simulink model "simu_gimbal"  (R2020a)
settings: Solver=FixedStepAuto  StartTime=0.0  StopTime=20  FixedStep=0.002  RelTol=1e-3
InitFcn:
  | init_conditions
values from neighbouring files (symbols this model uses):
  a = 1    [init_conditions.m]
  B = 0    [init_conditions.m]
  IB = diag([IBxy, IBxy, IBz])    [init_conditions.m]
  Iz = 3*(10^-5)    (= 3e-05)    [init_conditions.m]
  K = 0    [init_conditions.m]
  K1 = 800    [init_conditions.m]
  Lh = [0;0;0]    [init_conditions.m]
  m = (m_qc+0.006)*4 + m_main    (= 0.156)    [init_conditions.m]
  m_main = 0.012    [init_conditions.m]
undefined symbols (not defined in the file or in its folder): X, Y, Z
libraries: nesl_utility x25, sm_lib x24, sharedtransform x3, simulink x2
settings Model: Creator=Paul  LastModifiedBy=lee
settings DataIOCC: ReturnWorkspaceOutputs=off
settings DebuggingCC: ArithmeticOperatorsInVariantConditions=warning
settings SFSimCC: SimUseLocalCustomCode=off  CustomCodeUndefinedFunction=UseInterfaceOnly
settings RTWCC: RTWUseLocalCustomCode=off
settings ExplorerConfigSet: InternalSimMechanicsExplorerSettings="<ExplorerConfiguration><canonicalview>default</canonicalview><AnimationSetting><BasePlaybackSpeed>1.0</BasePlaybackSpeed><PlaybackSpeedFactor>1.0</PlaybackSpeedFactor></AnimationSetting><TilePanel><TileInfo><Tiles Columns=\"1\" Count=\"1\" Rows=\"1\"><Column Weight=\"1\"/><Row Weight=\"1\"/><Tile Height=\"1\" Width=\"1\" X=\"0\" Y=\"0\"/></Tiles></TileInfo><SceneInfo><SceneViewer><BGColor><R>0.60000002384185791</R><G>0.60000002384185791</G><B>0.60000002384185791</B></BGColor><Camera><DoPerspective>off</DoPerspective><Position><X>0.105450656144933763</X><Y>-0.11353615296204797</Y><Z>1.90562556726929944</Z></Position><Center><X>0.163716647023041978</X><Y>-0.0279701005319462764</Y><Z>-0.924535797346482835</Z></Center><Up><X>0.999736240990410918</X><Y>-0.0108255212991936745</Y><Z>0.0202547905189051844</Z></Up><ViewLimDist>1</ViewLimDist><YLim>0.670906463981186918</YLim><XLim>0.633335701998240408</XLim></Camera></SceneViewer></SceneInfo></TilePanel><MechEditorPanel><Cameras/><GfxPanelCameraMap/><VideoCreator><PlaybackSpeedRatio>1.0</PlaybackSpeedRatio><FrameRate>30</FrameRate><VideoFormat>Motion JPEG AVI</VideoFormat><FrameSize>auto</FrameSize></VideoCreator></MechEditorPanel></ExplorerConfiguration>"

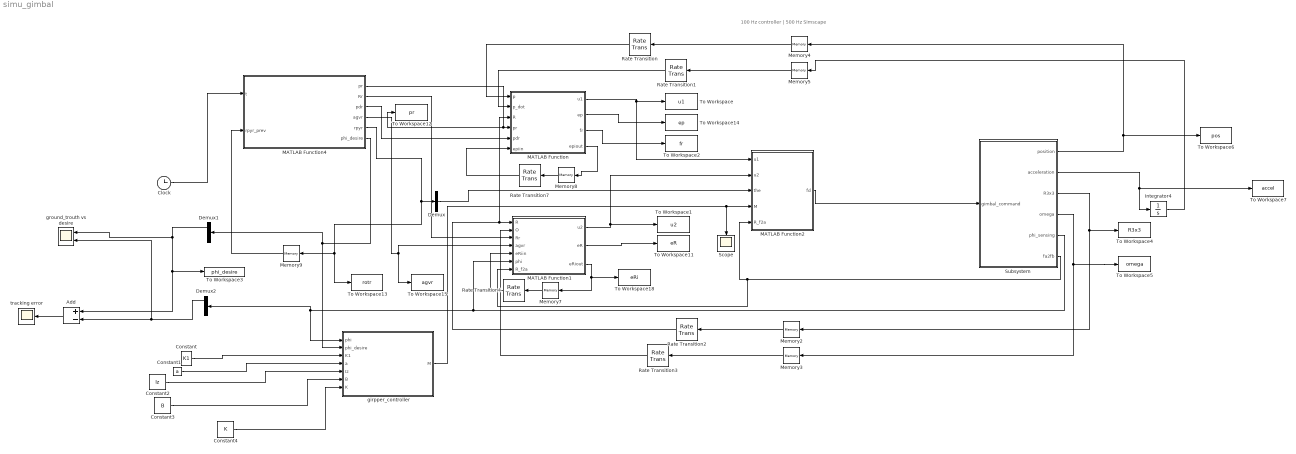
== system simu_gimbal ==
  note: 100 Hz controller | 500 Hz Simscape
  Add : Sum  Inputs=+-
  Clock : Clock
  Constant : Constant  Value=K1
  Constant1 : Constant  Value=a
  Constant2 : Constant  Value=Iz
  Constant3 : Constant  Value=B
  Constant4 : Constant  Value=K
  Demux : Demux  Outputs=3
  Demux1 : Demux  Outputs=3
  Demux2 : Demux  Outputs=3
  Integrator4 : Integrator  InitialCondition=[0;0;0]
  MATLAB Function : MATLAB Function  TreatAsAtomicUnit=on
  MATLAB Function1 : MATLAB Function  TreatAsAtomicUnit=on
  MATLAB Function2 : MATLAB Function  TreatAsAtomicUnit=on
  MATLAB Function4 : MATLAB Function  TreatAsAtomicUnit=on
  Memory2 : Memory  InitialCondition=eye(3)
  Memory{3..5,7..9} (6 alike) : Memory  InitialCondition=[0;0;0]
  Rate Transition{,1..4,7} (6 alike) : RateTransition  OutPortSampleTime=0.01
  Scope : Scope
  Subsystem : Subsystem
  To Workspace : ToWorkspace  VariableName=u1  SaveFormat=Timeseries  SampleTime=-1
  To Workspace1 : ToWorkspace  VariableName=u2  SaveFormat=Timeseries  SampleTime=-1
  To Workspace11 : ToWorkspace  VariableName=eR  SaveFormat=Timeseries  SampleTime=-1
  To Workspace12 : ToWorkspace  VariableName=pr  SaveFormat=Timeseries  SampleTime=-1
  To Workspace13 : ToWorkspace  VariableName=rotr  SaveFormat=Timeseries  SampleTime=-1
  To Workspace14 : ToWorkspace  VariableName=ep  SaveFormat=Timeseries  SampleTime=-1
  To Workspace15 : ToWorkspace  VariableName=agvr  SaveFormat=Timeseries  SampleTime=-1
  To Workspace18 : ToWorkspace  VariableName=eRi  SaveFormat=Timeseries  SampleTime=-1
  To Workspace2 : ToWorkspace  VariableName=fr  SaveFormat=Timeseries  SampleTime=-1
  To Workspace3 : ToWorkspace  VariableName=phi_desire  SaveFormat=Timeseries  SampleTime=-1
  To Workspace4 : ToWorkspace  VariableName=R3x3  SaveFormat=Timeseries  SampleTime=-1
  To Workspace5 : ToWorkspace  VariableName=omega  SaveFormat=Timeseries  SampleTime=-1
  To Workspace6 : ToWorkspace  VariableName=pos  SaveFormat=Timeseries  SampleTime=-1
  To Workspace7 : ToWorkspace  VariableName=accel  SaveFormat=Timeseries  SampleTime=-1
  girpper_controller : MATLAB Function  TreatAsAtomicUnit=on
  ground_trouth vs desire : Scope  NumInputPorts=2
  tracking error : Scope
  wires:
  MATLAB Function/1(u1) -> MATLAB Function2/1(u1), To Workspace/1
  MATLAB Function1/1(u2) -> MATLAB Function2/2(u2), To Workspace1/1
  Subsystem/3(R3x3) -> To Workspace4/1, Memory2/1
  Memory2/1 -> Rate Transition2/1
  Subsystem/4(omega) -> To Workspace5/1, Memory3/1
  Memory3/1 -> Rate Transition3/1
  Memory4/1 -> Rate Transition/1
  Memory5/1 -> Rate Transition1/1
  Subsystem/1(position) -> Memory4/1, To Workspace6/1
  Subsystem/2(acceleration) -> To Workspace7/1, Integrator4/1
  Integrator4/1 -> Memory5/1
  Clock/1 -> MATLAB Function4/1(t)
  MATLAB Function4/1(pr) -> To Workspace12/1, MATLAB Function/4(pr)
  MATLAB Function4/2(Rr) -> MATLAB Function1/3(Rr)
  MATLAB Function/3(fr) -> To Workspace2/1
  MATLAB Function2/1(fd) -> Subsystem/1(gimbal_command)
  MATLAB Function1/2(eR) -> To Workspace11/1
  MATLAB Function/2(ep) -> To Workspace14/1
  MATLAB Function1/3(eRiout) -> To Workspace18/1, Memory7/1
  Rate Transition/1 -> MATLAB Function/1(p)
  Rate Transition1/1 -> MATLAB Function/2(p_dot)
  Rate Transition2/1 -> MATLAB Function1/1(R), MATLAB Function/3(R)
  Rate Transition3/1 -> MATLAB Function1/2(O)
  Memory7/1 -> Rate Transition4/1
  Rate Transition4/1 -> MATLAB Function1/5(eRiin)
  Memory8/1 -> Rate Transition7/1
  MATLAB Function/4(epiout) -> Memory8/1
  Rate Transition7/1 -> MATLAB Function/6(epiin)
  MATLAB Function4/3(pdr) -> MATLAB Function/5(pdr)
  MATLAB Function4/4(agvr) -> To Workspace15/1, MATLAB Function1/4(agvr)
  MATLAB Function4/5(rpyr) -> To Workspace13/1, Memory9/1, Demux/1
  Memory9/1 -> MATLAB Function4/2(rpyr_prev)
  Demux/2 -> MATLAB Function2/3(the)
  Subsystem/5(phi_sensing) -> MATLAB Function1/6(phi), girpper_controller/1(phi), Demux2/1
  MATLAB Function4/6(phi_desire) -> Demux1/1, girpper_controller/2(phi_desire)
  Constant/1 -> girpper_controller/3(K1)
  Constant1/1 -> girpper_controller/4(a)
  girpper_controller/1(M) -> Scope/1, MATLAB Function2/4(M)
  Add/1 -> tracking error/1
  Demux1/1 -> To Workspace3/1, Add/1, ground_trouth vs desire/1
  Demux2/1 -> ground_trouth vs desire/2, Add/2
  Constant2/1 -> girpper_controller/5(Iz)
  Constant3/1 -> girpper_controller/6(B)
  Constant4/1 -> girpper_controller/7(K)
  Subsystem/6(fa2fb) -> MATLAB Function1/7(R_f2a), MATLAB Function2/5(R_f2a)

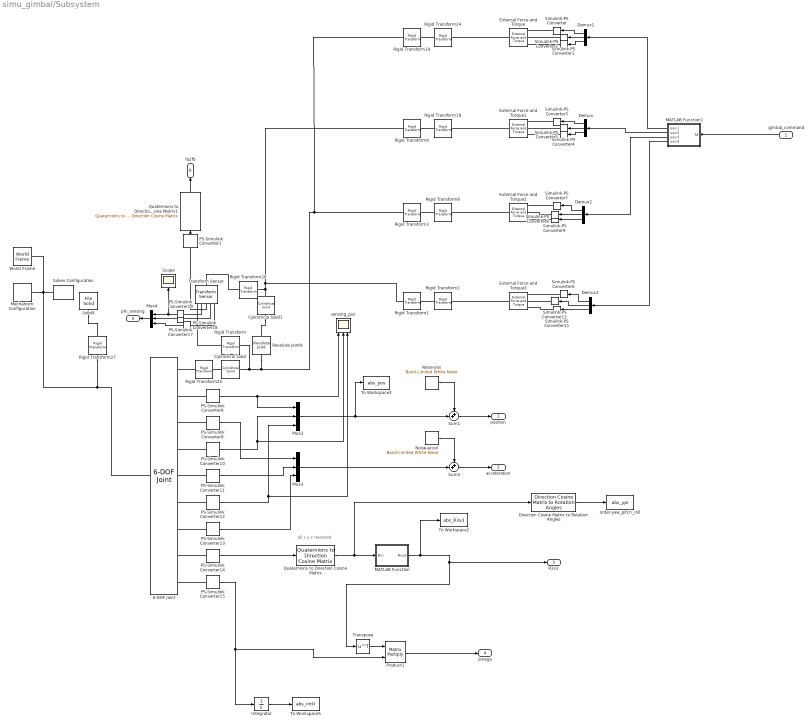
== system simu_gimbal/Subsystem ==
  note: all x y z reversed
  gimbal_command : Inport
  6-DOF Joint : sm_lib/Joints/6-DOF Joint  JointMode=Normal  SenseConstraintForce=off  SenseConstraintForceX=off  SenseConstraintForceY=off  SenseConstraintForceZ=off  SenseConstraintTorque=off  SenseConstraintTorqueX=off  SenseConstraintTorqueY=off  SenseConstraintTorqueZ=off  SenseTotalForce=off  SenseTotalForceX=off  SenseTotalForceY=off  SenseTotalForceZ=off  SenseTotalTorque=off  SenseTotalTorqueX=off  SenseTotalTorqueY=off  SenseTotalTorqueZ=off  CompositeWrenchDir=FollowerOnBase  CompositeWrenchFrame=BaseFrame  PxEquilibriumPosition=0  PxEquilibriumPositionUnits=m  PxSpringStiffness=0  PxSpringStiffnessUnits=N/m  PxDampingCoefficient=0  PxDampingCoefficientUnits=N/(m/s)  PxTorqueActuationMode=NoTorque  PxMotionActuationMode=ComputedMotion  PxSensePosition=on  PxSenseVelocity=off  PxSenseAcceleration=on  PxSenseTorqueForce=off  PxSenseLowerLimitTorqueForce=off  PxSenseUpperLimitTorqueForce=off  PxLowerLimitSpecify=off  PxLowerLimitBound=-1  PxLowerLimitBoundUnits=m  PxLowerLimitStiffness=1e6  PxLowerLimitStiffnessUnits=N/m  PxLowerLimitDamping=1e3  PxLowerLimitDampingUnits=N/(m/s)  PxLowerLimitTransitionRegionWidth=1e-4  PxLowerLimitTransitionRegionWidthUnits=m  PxUpperLimitSpecify=off  PxUpperLimitBound=1  PxUpperLimitBoundUnits=m  PxUpperLimitStiffness=1e6  PxUpperLimitStiffnessUnits=N/m  PxUpperLimitDamping=1e3  PxUpperLimitDampingUnits=N/(m/s)  PxUpperLimitTransitionRegionWidth=1e-4  PxUpperLimitTransitionRegionWidthUnits=m  PxPositionTargetSpecify=off  PxPositionTargetPriority=High  PxPositionTargetValue=0  PxPositionTargetValueUnits=m  PxVelocityTargetSpecify=off  PxVelocityTargetPriority=High  PxVelocityTargetValue=0  PxVelocityTargetValueUnits=m/s  PyEquilibriumPosition=0  PyEquilibriumPositionUnits=m  PySpringStiffness=0  PySpringStiffnessUnits=N/m  PyDampingCoefficient=0  PyDampingCoefficientUnits=N/(m/s)  PyTorqueActuationMode=NoTorque  PyMotionActuationMode=ComputedMotion  PySensePosition=on  PySenseVelocity=off  PySenseAcceleration=on  PySenseTorqueForce=off  PySenseLowerLimitTorqueForce=off  PySenseUpperLimitTorqueForce=off  PyLowerLimitSpecify=off  PyLowerLimitBound=-1  PyLowerLimitBoundUnits=m  PyLowerLimitStiffness=1e6  PyLowerLimitStiffnessUnits=N/m  PyLowerLimitDamping=1e3  PyLowerLimitDampingUnits=N/(m/s)  PyLowerLimitTransitionRegionWidth=1e-4  PyLowerLimitTransitionRegionWidthUnits=m  PyUpperLimitSpecify=off  PyUpperLimitBound=1  PyUpperLimitBoundUnits=m  PyUpperLimitStiffness=1e6  PyUpperLimitStiffnessUnits=N/m  PyUpperLimitDamping=1e3  PyUpperLimitDampingUnits=N/(m/s)  PyUpperLimitTransitionRegionWidth=1e-4  PyUpperLimitTransitionRegionWidthUnits=m  PyPositionTargetSpecify=off  PyPositionTargetPriority=High  PyPositionTargetValue=0  PyPositionTargetValueUnits=m  PyVelocityTargetSpecify=off  PyVelocityTargetPriority=High  PyVelocityTargetValue=0  PyVelocityTargetValueUnits=m/s  PzEquilibriumPosition=0  PzEquilibriumPositionUnits=m  PzSpringStiffness=0  PzSpringStiffnessUnits=N/m  PzDampingCoefficient=0  PzDampingCoefficientUnits=N/(m/s)  PzTorqueActuationMode=NoTorque  PzMotionActuationMode=ComputedMotion  PzSensePosition=on  PzSenseVelocity=off  PzSenseAcceleration=on  PzSenseTorqueForce=off  PzSenseLowerLimitTorqueForce=off  PzSenseUpperLimitTorqueForce=off  PzLowerLimitSpecify=off  PzLowerLimitBound=-1  PzLowerLimitBoundUnits=m  PzLowerLimitStiffness=1e6  PzLowerLimitStiffnessUnits=N/m  PzLowerLimitDamping=1e3  PzLowerLimitDampingUnits=N/(m/s)  PzLowerLimitTransitionRegionWidth=1e-4  PzLowerLimitTransitionRegionWidthUnits=m  PzUpperLimitSpecify=off  PzUpperLimitBound=1  PzUpperLimitBoundUnits=m  PzUpperLimitStiffness=1e6  PzUpperLimitStiffnessUnits=N/m  PzUpperLimitDamping=1e3  PzUpperLimitDampingUnits=N/(m/s)  PzUpperLimitTransitionRegionWidth=1e-4  PzUpperLimitTransitionRegionWidthUnits=m  PzPositionTargetSpecify=off  PzPositionTargetPriority=High  PzPositionTargetValue=0  PzPositionTargetValueUnits=m  PzVelocityTargetSpecify=off  PzVelocityTargetPriority=High  PzVelocityTargetValue=0  PzVelocityTargetValueUnits=m/s  SphDefPosRotationMethod=None  SphDefPosRotationAngleUnits=deg  SphDefPosRotationStandardAxis=+Z  SphDefPosRotationAngle=0.0  SphDefPosRotationArbitraryAxis=[0 0 1]  SphDefPosFollAlignAxisA=+X  SphDefPosBaseAlignAxisA=+Y  SphDefPosFollAlignAxisB=+Y  SphDefPosBaseAlignAxisB=+Z  SphDefPosRotationSequenceAxes=FollowerAxes  SphDefPosRotationSequence=XYX  SphDefPosRotationSequenceAngles=[0 0 0]  SphDefPosRotationSequenceAnglesUnits=deg  SphDefPosRotationMatrix=[1 0 0; 0 1 0; 0 0 1]  SphEqPosRotationMethod=None  SphEqPosRotationAngleUnits=deg  SphEqPosRotationStandardAxis=+Z  SphEqPosRotationAngle=0.0  SphEqPosRotationArbitraryAxis=[0 0 1]  SphEqPosFollAlignAxisA=+X  SphEqPosBaseAlignAxisA=+Y  SphEqPosFollAlignAxisB=+Y  SphEqPosBaseAlignAxisB=+Z  SphEqPosRotationSequenceAxes=FollowerAxes  SphEqPosRotationSequence=XYX  SphEqPosRotationSequenceAngles=[0 0 0]  SphEqPosRotationSequenceAnglesUnits=deg  SphEqPosRotationMatrix=[1 0 0; 0 1 0; 0 0 1]  SphSpringStiffness=0  SphSpringStiffnessUnits=N*m/deg  SphDampingCoefficient=0  SphDampingCoefficientUnits=N*m/(deg/s)  SphActuateTorqueX=off  SphActuateTorqueY=off  SphActuateTorqueZ=off  SphActuateTorque=off  SphTorqueActuationMode=NoTorque  SphMotionActuationMode=ComputedMotion  SphActuationFrame=BaseFrame  SphSensePosition=on  SphSenseVelocityX=off  SphSenseVelocityY=off  SphSenseVelocityZ=off  SphSenseVelocity=on  SphSenseAccelerationX=off  SphSenseAccelerationY=off  SphSenseAccelerationZ=off  SphSenseAcceleration=off  SphSenseTorqueX=off  SphSenseTorqueY=off  SphSenseTorqueZ=off  SphSenseTorqueForce=off  SphSenseLowerLimitTorqueMag=off  SphSenseUpperLimitTorqueMag=off  SphSensingFrame=BaseFrame  SphLowerLimitSpecify=off  SphLowerLimitBound=15  SphLowerLimitBoundUnits=deg  SphLowerLimitStiffness=1e4  SphLowerLimitStiffnessUnits=N*m/deg  SphLowerLimitDamping=10  SphLowerLimitDampingUnits=N*m/(deg/s)  SphLowerLimitTransitionRegionWidth=0.1  SphLowerLimitTransitionRegionWidthUnits=deg  SphUpperLimitSpecify=off  SphUpperLimitBound=45  SphUpperLimitBoundUnits=deg  SphUpperLimitStiffness=1e4  SphUpperLimitStiffnessUnits=N*m/deg  SphUpperLimitDamping=10  SphUpperLimitDampingUnits=N*m/(deg/s)  SphUpperLimitTransitionRegionWidth=0.1  SphUpperLimitTransitionRegionWidthUnits=deg  SphPositionTargetRotationMethod=None  SphPositionTargetRotationAngleUnits=deg  SphPositionTargetRotationStandardAxis=+Z  SphPositionTargetRotationAngle=0.0  SphPositionTargetRotationArbitraryAxis=[0 0 1]  SphPositionTargetFollAlignAxisA=+X  SphPositionTargetBaseAlignAxisA=+Y  SphPositionTargetFollAlignAxisB=+Y  SphPositionTargetBaseAlignAxisB=+Z  SphPositionTargetRotationSequenceAxes=FollowerAxes  SphPositionTargetRotationSequence=XYX  SphPositionTargetRotationSequenceAngles=[0 0 0]  SphPositionTargetRotationSequenceAnglesUnits=deg  SphPositionTargetRotationMatrix=[1 0 0; 0 1 0; 0 0 1]  SphPositionTargetSpecify=off  SphPositionTargetPriority=High  SphVelocityTargetValue=[0 0 0]  SphVelocityTargetValueUnits=deg/s  SphVelocityTargetSpecify=off  SphVelocityTargetPriority=High  SphVelocityTargetInFollowerFrame=on
  Cylindrical Solid : sm_lib/Body Elements/Cylindrical Solid  GraphicAmbientColor=[0.15 0.15 0.15 1.0]  BasedOnType=Density  CenterOfMass=[0 0 0]  CenterOfMassUnits=m  GraphicDiffuseColor=[0.5 0.5 0.5]  CylinderLength=300  CylinderLengthUnits=mm  CylinderRadius=3  CylinderRadiusUnits=mm  Density=1000  DensityUnits=kg/m^3  DoExposeReferenceFrame=off  GraphicEmissiveColor=[0.0 0.0 0.0 1.0]  ExportEntireGeometry=off  SerializedFrames=<Frames><Frame><Id>Frame1</Id><Value><Name>F1</Name><Origin><Source>ReferenceFrame</Source><FeatureName></FeatureName></Origin><PrimaryAxis><DefinedDirection>+Z</DefinedDirection><Source>ReferenceFrame</Source><SourceDirection>+Y</SourceDirection><FeatureName></FeatureName></PrimaryAxis><SecondaryAxis><DefinedDirection>+Y</DefinedDirection><Source>ReferenceFrame</Source><SourceDirection>+X</SourceDirection><FeatureName></FeatureName></SecondaryAxis></Value></Frame><Frame><Id>Frame2</Id><Value><Name>F2</Name><Origin><Source>ReferenceFrame</Source><FeatureName></FeatureName></Origin><PrimaryAxis><DefinedDirection>+Z</DefinedDirection><Source>ReferenceFrame</Source><SourceDirection>+Y</SourceDirection><FeatureName></FeatureName></PrimaryAxis><SecondaryAxis><DefinedDirection>+Y</DefinedDirection><Source>ReferenceFrame</Source><SourceDirection>+X</SourceDirection><FeatureName></FeatureName></SecondaryAxis></Value></Frame></Frames>  MarkerShape=Sphere  MarkerSize=10  GraphicType=FromGeometry  InertiaType=Custom  Mass=m_main/2  MassUnits=kg  MomentsOfInertia=[3e-5 3e-5 3e-5]  MomentsOfInertiaUnits=kg*m^2  GraphicOpacity=1.0  ProductsOfInertia=[0 0 0]  ProductsOfInertiaUnits=kg*m^2  GraphicShininess=75  GraphicSpecularColor=[0.5 0.5 0.5 1.0]  GraphicVisPropType=SimpleVisualProperties
  Cylindrical Solid1 : sm_lib/Body Elements/Cylindrical Solid  GraphicAmbientColor=[0.15 0.15 0.15 1.0]  BasedOnType=Density  CenterOfMass=[0 0 0]  CenterOfMassUnits=m  GraphicDiffuseColor=[0.5 0.5 0.5]  CylinderLength=300  CylinderLengthUnits=mm  CylinderRadius=3  CylinderRadiusUnits=mm  Density=1000  DensityUnits=kg/m^3  DoExposeReferenceFrame=off  GraphicEmissiveColor=[0.0 0.0 0.0 1.0]  ExportEntireGeometry=off  SerializedFrames=<Frames><Frame><Id>Frame1</Id><Value><Name>F1</Name><Origin><Source>ReferenceFrame</Source><FeatureName></FeatureName></Origin><PrimaryAxis><DefinedDirection>+Z</DefinedDirection><Source>ReferenceFrame</Source><SourceDirection>+Y</SourceDirection><FeatureName></FeatureName></PrimaryAxis><SecondaryAxis><DefinedDirection>+Y</DefinedDirection><Source>ReferenceFrame</Source><SourceDirection>+Z</SourceDirection><FeatureName></FeatureName></SecondaryAxis></Value></Frame><Frame><Id>Frame2</Id><Value><Name>F2</Name><Origin><Source>ReferenceFrame</Source><FeatureName></FeatureName></Origin><PrimaryAxis><DefinedDirection>+Z</DefinedDirection><Source>ReferenceFrame</Source><SourceDirection>+Y</SourceDirection><FeatureName></FeatureName></PrimaryAxis><SecondaryAxis><DefinedDirection>+Y</DefinedDirection><Source>ReferenceFrame</Source><SourceDirection>+Z</SourceDirection><FeatureName></FeatureName></SecondaryAxis></Value></Frame></Frames>  MarkerShape=Sphere  MarkerSize=10  GraphicType=FromGeometry  InertiaType=Custom  Mass=m_main/2  MassUnits=kg  MomentsOfInertia=[3e-5 3e-5 3e-5]  MomentsOfInertiaUnits=kg*m^2  GraphicOpacity=1.0  ProductsOfInertia=[0 0 0]  ProductsOfInertiaUnits=kg*m^2  GraphicShininess=75  GraphicSpecularColor=[0.5 0.5 0.5 1.0]  GraphicVisPropType=SimpleVisualProperties
  Demux{,1..3} (4 alike) : Demux  Outputs=3
  Direction Cosine Matrix to Rotation Angles : sharedtransform/Direction Cosine Matrix to Rotation Angles  rotationOrder=ZYX  aMode=aMode  action=None  tolerance=eps(2)
      settings: SourceProductBaseCode=AE,PW,MT,VE,VP
  External Force and Torque{,1..3} (4 alike) : sm_lib/Forces and Torques/External Force and Torque  ForceResolutionFrame=AttachedFrame  EnableForceX=on  EnableForceY=on  EnableForceZ=on  EnableForce=off  TorqueResolutionFrame=AttachedFrame  EnableTorqueX=off  EnableTorqueY=off  EnableTorqueZ=off  EnableTorque=off
  Integrator : Integrator
  MATLAB Function : MATLAB Function  TreatAsAtomicUnit=on
  MATLAB Function1 : MATLAB Function  TreatAsAtomicUnit=on
  Mechanism Configuration : sm_lib/Utilities/Mechanism Configuration  UniformGravity=Constant  GravityVector=[0 0 -9.81]  GravityUnits=m/s^2  LinearizationDelta=0.002
  Mux2 : Mux  Inputs=3
  Mux3 : Mux  Inputs=3
  Mux4 : Mux  Inputs=3
  Noise-accel : simulink/Sources/Band-Limited White Noise  Cov=1e-8*[1;1;1]  Ts=0.002  seed=[51521; 65486; 13464]
  Noise-pos : simulink/Sources/Band-Limited White Noise  Cov=3e-9*[1;1;1]  Ts=0.002  seed=[35624; 14890; 47463]
  PS-Simulink Converter{1,8..15} (9 alike) : nesl_utility/PS-Simulink Converter  PhysicalDomain=network_engine_domain  SubClassName=ps_output  LeftPortType=input  RightPortType=output  PseudoPeriodic=off  Frequencies=[]  Unit=1  AffineConversion=off
  PS-Simulink Converter17 : nesl_utility/PS-Simulink Converter  PhysicalDomain=network_engine_domain  SubClassName=ps_output  LeftPortType=input  RightPortType=output  PseudoPeriodic=off  Frequencies=[]  Unit=inherit  AffineConversion=off
  PS-Simulink Converter18 : nesl_utility/PS-Simulink Converter  PhysicalDomain=network_engine_domain  SubClassName=ps_output  LeftPortType=input  RightPortType=output  PseudoPeriodic=off  Frequencies=[]  Unit=inherit  AffineConversion=off
  PS-Simulink Converter19 : nesl_utility/PS-Simulink Converter  PhysicalDomain=network_engine_domain  SubClassName=ps_output  LeftPortType=input  RightPortType=output  PseudoPeriodic=off  Frequencies=[]  Unit=inherit  AffineConversion=off
  Product1 : Product  Multiplication=Matrix(*)
  Quaternions to Direction Cosine Matrix : sharedtransform/Quaternions to  Direction Cosine Matrix  aMode=aMode
      settings: SourceProductBaseCode=AE,PW,MT,VE,VP
  Quaternions to Direction Cosine Matrix1 : sharedtransform/Quaternions to  Direction Cosine Matrix  aMode=aMode
      settings: SourceProductBaseCode=AE,PW,MT,VE,VP
  Revolute Joint9 : sm_lib/Joints/Revolute Joint  JointMode=Normal  SenseConstraintForce=off  SenseConstraintForceX=off  SenseConstraintForceY=off  SenseConstraintForceZ=off  SenseConstraintTorque=off  SenseConstraintTorqueX=off  SenseConstraintTorqueY=off  SenseConstraintTorqueZ=off  SenseTotalForce=off  SenseTotalForceX=off  SenseTotalForceY=off  SenseTotalForceZ=off  SenseTotalTorque=off  SenseTotalTorqueX=off  SenseTotalTorqueY=off  SenseTotalTorqueZ=off  CompositeWrenchDir=FollowerOnBase  CompositeWrenchFrame=BaseFrame  EquilibriumPosition=0  EquilibriumPositionUnits=deg  SpringStiffness=0  SpringStiffnessUnits=N*m/deg  DampingCoefficient=0  DampingCoefficientUnits=N*m/(deg/s)  TorqueActuationMode=NoTorque  MotionActuationMode=ComputedMotion  SensePosition=off  SenseVelocity=off  SenseAcceleration=off  SenseTorqueForce=off  SenseLowerLimitTorqueForce=off  SenseUpperLimitTorqueForce=off  LowerLimitSpecify=off  LowerLimitBound=-90  LowerLimitBoundUnits=deg  LowerLimitStiffness=1e4  LowerLimitStiffnessUnits=N*m/deg  LowerLimitDamping=10  LowerLimitDampingUnits=N*m/(deg/s)  LowerLimitTransitionRegionWidth=0.1  LowerLimitTransitionRegionWidthUnits=deg  UpperLimitSpecify=off  UpperLimitBound=90  UpperLimitBoundUnits=deg  UpperLimitStiffness=1e4  UpperLimitStiffnessUnits=N*m/deg  UpperLimitDamping=10  UpperLimitDampingUnits=N*m/(deg/s)  UpperLimitTransitionRegionWidth=0.1  UpperLimitTransitionRegionWidthUnits=deg  PositionTargetSpecify=off  PositionTargetPriority=High  PositionTargetValue=0  PositionTargetValueUnits=deg  VelocityTargetSpecify=off  VelocityTargetPriority=High  VelocityTargetValue=0  VelocityTargetValueUnits=deg/s
  Rigid Transform : sm_lib/Frames and Transforms/Rigid Transform  TranslationMethod=None  TranslationStandardOffset=0  TranslationLengthUnit=m  TranslationStandardAxis=+Z  TranslationCartesianOffset=[0 0 0]  TranslationROffset=0  TranslationROffsetUnits=m  TranslationZOffset=0  TranslationZOffsetUnits=m  TranslationThetaOffset=0  TranslationThetaOffsetUnits=deg  RotationMethod=StandardAxis  RotationAngleUnits=deg  RotationStandardAxis=+Z  RotationAngle=90  RotationArbitraryAxis=[0 0 1]  FollAlignAxisA=+X  BaseAlignAxisA=+Y  FollAlignAxisB=+Y  BaseAlignAxisB=+Z  RotationSequenceAxes=FollowerAxes  RotationSequence=XYX  RotationSequenceAngles=[0 0 0]  RotationSequenceAnglesUnits=deg  RotationMatrix=[1 0 0; 0 1 0; 0 0 1]
  Rigid Transform1 : sm_lib/Frames and Transforms/Rigid Transform  TranslationMethod=None  TranslationStandardOffset=0  TranslationLengthUnit=m  TranslationStandardAxis=+Z  TranslationCartesianOffset=[0 0 0]  TranslationROffset=0  TranslationROffsetUnits=m  TranslationZOffset=0  TranslationZOffsetUnits=m  TranslationThetaOffset=0  TranslationThetaOffsetUnits=deg  RotationMethod=StandardAxis  RotationAngleUnits=deg  RotationStandardAxis=+Z  RotationAngle=270  RotationArbitraryAxis=[0 0 1]  FollAlignAxisA=+X  BaseAlignAxisA=+Y  FollAlignAxisB=+Y  BaseAlignAxisB=+Z  RotationSequenceAxes=FollowerAxes  RotationSequence=XYX  RotationSequenceAngles=[0 0 0]  RotationSequenceAnglesUnits=deg  RotationMatrix=[1 0 0; 0 1 0; 0 0 1]
  Rigid Transform{2,8,18,24} (4 alike) : sm_lib/Frames and Transforms/Rigid Transform  TranslationMethod=StandardAxis  TranslationStandardOffset=0.18  TranslationLengthUnit=m  TranslationStandardAxis=+X  TranslationCartesianOffset=[0 0 0]  TranslationROffset=0  TranslationROffsetUnits=m  TranslationZOffset=0  TranslationZOffsetUnits=m  TranslationThetaOffset=0  TranslationThetaOffsetUnits=deg  RotationMethod=None  RotationAngleUnits=deg  RotationStandardAxis=+Z  RotationAngle=0.0  RotationArbitraryAxis=[0 0 1]  FollAlignAxisA=+X  BaseAlignAxisA=+Y  FollAlignAxisB=+Y  BaseAlignAxisB=+Z  RotationSequenceAxes=FollowerAxes  RotationSequence=XYX  RotationSequenceAngles=[0 0 0]  RotationSequenceAnglesUnits=deg  RotationMatrix=[1 0 0; 0 1 0; 0 0 1]
  Rigid Transform19 : sm_lib/Frames and Transforms/Rigid Transform  TranslationMethod=None  TranslationStandardOffset=0  TranslationLengthUnit=m  TranslationStandardAxis=+Z  TranslationCartesianOffset=[0 0 0]  TranslationROffset=0  TranslationROffsetUnits=m  TranslationZOffset=0  TranslationZOffsetUnits=m  TranslationThetaOffset=0  TranslationThetaOffsetUnits=deg  RotationMethod=StandardAxis  RotationAngleUnits=deg  RotationStandardAxis=+Z  RotationAngle=0  RotationArbitraryAxis=[0 0 1]  FollAlignAxisA=+X  BaseAlignAxisA=+Y  FollAlignAxisB=+Y  BaseAlignAxisB=+Z  RotationSequenceAxes=FollowerAxes  RotationSequence=XYX  RotationSequenceAngles=[0 0 0]  RotationSequenceAnglesUnits=deg  RotationMatrix=[1 0 0; 0 1 0; 0 0 1]
  Rigid Transform25 : sm_lib/Frames and Transforms/Rigid Transform  TranslationMethod=None  TranslationStandardOffset=0  TranslationLengthUnit=m  TranslationStandardAxis=-Z  TranslationCartesianOffset=[0 0 0]  TranslationROffset=0  TranslationROffsetUnits=m  TranslationZOffset=0  TranslationZOffsetUnits=m  TranslationThetaOffset=0  TranslationThetaOffsetUnits=deg  RotationMethod=None  RotationAngleUnits=deg  RotationStandardAxis=+Z  RotationAngle=270  RotationArbitraryAxis=[0 0 1]  FollAlignAxisA=+X  BaseAlignAxisA=+Y  FollAlignAxisB=+Y  BaseAlignAxisB=+Z  RotationSequenceAxes=FollowerAxes  RotationSequence=XYX  RotationSequenceAngles=[0 0 0]  RotationSequenceAnglesUnits=deg  RotationMatrix=[1 0 0; 0 1 0; 0 0 1]
  Rigid Transform26 : sm_lib/Frames and Transforms/Rigid Transform  TranslationMethod=None  TranslationStandardOffset=0  TranslationLengthUnit=m  TranslationStandardAxis=+Z  TranslationCartesianOffset=[0 0 0]  TranslationROffset=0  TranslationROffsetUnits=m  TranslationZOffset=0  TranslationZOffsetUnits=m  TranslationThetaOffset=0  TranslationThetaOffsetUnits=deg  RotationMethod=None  RotationAngleUnits=deg  RotationStandardAxis=+Z  RotationAngle=90  RotationArbitraryAxis=[0 0 1]  FollAlignAxisA=+X  BaseAlignAxisA=+Y  FollAlignAxisB=+Y  BaseAlignAxisB=+Z  RotationSequenceAxes=FollowerAxes  RotationSequence=XYX  RotationSequenceAngles=[0 0 0]  RotationSequenceAnglesUnits=deg  RotationMatrix=[1 0 0; 0 1 0; 0 0 1]
  Rigid Transform27 : sm_lib/Frames and Transforms/Rigid Transform  TranslationMethod=StandardAxis  TranslationStandardOffset=0.5  TranslationLengthUnit=m  TranslationStandardAxis=+Y  TranslationCartesianOffset=[0 0 0]  TranslationROffset=0  TranslationROffsetUnits=m  TranslationZOffset=0  TranslationZOffsetUnits=m  TranslationThetaOffset=0  TranslationThetaOffsetUnits=deg  RotationMethod=None  RotationAngleUnits=deg  RotationStandardAxis=+Z  RotationAngle=0.0  RotationArbitraryAxis=[0 0 1]  FollAlignAxisA=+X  BaseAlignAxisA=+Y  FollAlignAxisB=+Y  BaseAlignAxisB=+Z  RotationSequenceAxes=FollowerAxes  RotationSequence=XYX  RotationSequenceAngles=[0 0 0]  RotationSequenceAnglesUnits=deg  RotationMatrix=[1 0 0; 0 1 0; 0 0 1]
  Rigid Transform3 : sm_lib/Frames and Transforms/Rigid Transform  TranslationMethod=None  TranslationStandardOffset=0  TranslationLengthUnit=m  TranslationStandardAxis=+Z  TranslationCartesianOffset=[0 0 0]  TranslationROffset=0  TranslationROffsetUnits=m  TranslationZOffset=0  TranslationZOffsetUnits=m  TranslationThetaOffset=0  TranslationThetaOffsetUnits=deg  RotationMethod=StandardAxis  RotationAngleUnits=deg  RotationStandardAxis=+Z  RotationAngle=180  RotationArbitraryAxis=[0 0 1]  FollAlignAxisA=+X  BaseAlignAxisA=+Y  FollAlignAxisB=+Y  BaseAlignAxisB=+Z  RotationSequenceAxes=FollowerAxes  RotationSequence=XYX  RotationSequenceAngles=[0 0 0]  RotationSequenceAnglesUnits=deg  RotationMatrix=[1 0 0; 0 1 0; 0 0 1]
  Rigid Transform9 : sm_lib/Frames and Transforms/Rigid Transform  TranslationMethod=None  TranslationStandardOffset=0  TranslationLengthUnit=m  TranslationStandardAxis=+Z  TranslationCartesianOffset=[0 0 0]  TranslationROffset=0  TranslationROffsetUnits=m  TranslationZOffset=0  TranslationZOffsetUnits=m  TranslationThetaOffset=0  TranslationThetaOffsetUnits=deg  RotationMethod=StandardAxis  RotationAngleUnits=deg  RotationStandardAxis=+Z  RotationAngle=90  RotationArbitraryAxis=[0 0 1]  FollAlignAxisA=+X  BaseAlignAxisA=+Y  FollAlignAxisB=+Y  BaseAlignAxisB=+Z  RotationSequenceAxes=FollowerAxes  RotationSequence=XYX  RotationSequenceAngles=[0 0 0]  RotationSequenceAnglesUnits=deg  RotationMatrix=[1 0 0; 0 1 0; 0 0 1]
  Scope : Scope
  Simulink-PS Converter{,1..9,11..12} (12 alike) : nesl_utility/Simulink-PS Converter  PhysicalDomain=network_engine_domain  SubClassName=ps_input  LeftPortType=input  RightPortType=output  PseudoPeriodic=off  Frequencies=[]  NoiseDistribution=none  NoiseParameters=[]  Unit=1  AffineConversion=off  FilteringAndDerivatives=provide  SimscapeFilterOrder=1  InputFilterTimeConstant=0.001  UdotUserProvided=0
  Solid9 : sm_lib/Body Elements/File Solid  ExtGeomFileName=/home/lee/workspace/matlab/2020a/ucla_gimbal/Gimbal_Platform_Simulation-main/circle_traj.STEP  UnitType=FromFile  ExtGeomFileUnits=m  StepReaderType=HEX  ExportConvexHullGeometry=off  InertiaType=Custom  Mass=m_main  MassUnits=kg  CenterOfMass=[0 0 0]  CenterOfMassUnits=m  MomentsOfInertia=[3e-5 3e-5 6e-5]  MomentsOfInertiaUnits=kg*m^2  ProductsOfInertia=[0 0 0]  ProductsOfInertiaUnits=kg*m^2  BasedOnType=Density  Density=1000  DensityUnits=kg/m^3  DoExposeReferenceFrame=on  SerializedFrames=<Frames/>  GraphicType=FromGeometry  MarkerShape=Sphere  MarkerSize=10  GraphicVisPropType=SimpleVisualProperties  GraphicDiffuseColor=[0.4 1.0 0.0]  GraphicSpecularColor=[0.5 0.5 0.5 1.0]  GraphicAmbientColor=[0.15 0.15 0.15 1.0]  GraphicEmissiveColor=[0.0 0.0 0.0 1.0]  GraphicShininess=75  GraphicOpacity=1.0
  Solver Configuration : nesl_utility/Solver Configuration  PhysicalDomain=network_engine_domain  SubClassName=solver  LeftPortType=input  RightPortType=generic  Tones=[]  Harmonics=[]  SimulateNoise=off  Profile=off  UseLocalSampling=off  EnableSwitchedLinearOptims=on  FrequencyDomain=off  UseCCode=off  RelTol=0.001  AbsTol=1e-06  MinStep=1e-09  ToWorkspace=off  RevertToSquareIcSolve=off  NumHomotopyIterations=100  PhasorMode=off  PhasorModeNumHarmonics=1  DoDC=off  ResidualTolerance=1e-09  UseLocalSolver=off  LocalSolverChoice=NE_BACKWARD_EULER_ADVANCER  LocalSolverSampleTime=0.001  DoFixedCost=off  MaxNonlinIter=3  MaxModeIter=2  LinearAlgebra=Sparse  EquationFormulation=NE_TIME_EF  DelaysMemoryBudget=1024  AutomaticFiltering=on  FilteringTimeConstant=0.002  PartitionStorageMethod=AS_NEEDED  PartitionMemoryBudget=1024  PartitionMethod=FAST
  Sum1 : Sum  Inputs=++|
  Sum2 : Sum  Inputs=++|
  To Workspace2 : ToWorkspace  VariableName=abs_R3x3  SaveFormat=Timeseries  SampleTime=-1
  To Workspace3 : ToWorkspace  VariableName=abs_pos  SaveFormat=Timeseries  SampleTime=-1
  To Workspace5 : ToWorkspace  VariableName=abs_intO  SaveFormat=Timeseries  SampleTime=-1
  Transform Sensor : sm_lib/Frames and Transforms/Transform Sensor  MeasurementFrame=Base  SenseAngle=on  SenseAxis=off  SenseAngle1=off  SenseAngle2=off  SenseAngle3=off  SenseQ=on  SenseR=off  SenseOmegaX=off  SenseOmegaY=off  SenseOmegaZ=on  SenseOmega1=off  SenseOmega2=off  SenseOmega3=off  SenseQDot=off  SenseRDot=off  SenseAlphaX=off  SenseAlphaY=off  SenseAlphaZ=on  SenseAlpha1=off  SenseAlpha2=off  SenseAlpha3=off  SenseQDDot=off  SenseRDDot=off  SenseX=off  SenseY=off  SenseZ=off  SenseRad=off  SenseAzim=off  SenseDist=off  SenseInc=off  SenseXDot=off  SenseYDot=off  SenseZDot=off  SenseRadDot=off  SenseAzimDot=off  SenseDistDot=off  SenseIncDot=off  SenseXDDot=off  SenseYDDot=off  SenseZDDot=off  SenseRadDDot=off  SenseAzimDDot=off  SenseDistDDot=off  SenseIncDDot=off
  Transpose : Math  Operator=transpose  SaturateOnIntegerOverflow=on
  World Frame : sm_lib/Frames and Transforms/World Frame
  order-yaw_pitch_roll : ToWorkspace  VariableName=abs_ypr  SaveFormat=Timeseries  SampleTime=-1
  sensing_pos : Scope  NumInputPorts=3
  position : Outport  VectorParamsAs1DForOutWhenUnconnected=off
  acceleration : Outport  Port=2  VectorParamsAs1DForOutWhenUnconnected=off
  R3x3 : Outport  Port=3  VectorParamsAs1DForOutWhenUnconnected=off
  omega : Outport  Port=4  VectorParamsAs1DForOutWhenUnconnected=off
  phi_sensing : Outport  Port=5
  fa2fb : Outport  Port=6
  wires:
  Quaternions to Direction Cosine Matrix/1 -> Direction Cosine Matrix to Rotation Angles/1, MATLAB Function/1(Rin)
  PS-Simulink Converter8/1 -> sensing_pos/1, Mux2/1
  PS-Simulink Converter10/1 -> sensing_pos/2, Mux2/2
  PS-Simulink Converter12/1 -> sensing_pos/3, Mux2/3
  PS-Simulink Converter9/1 -> Mux3/1
  PS-Simulink Converter11/1 -> Mux3/2
  PS-Simulink Converter13/1 -> Mux3/3
  PS-Simulink Converter15/1 -> Product1/2, Integrator/1
  Product1/1 -> omega/1
  MATLAB Function/1(Rout) -> To Workspace2/1, R3x3/1, Transpose/1
  Mux2/1 -> To Workspace3/1, Sum1/2
  Sum1/1 -> position/1
  Noise-pos/1 -> Sum1/1
  Mux3/1 -> Sum2/2
  Sum2/1 -> acceleration/1
  Noise-accel/1 -> Sum2/1
  Integrator/1 -> To Workspace5/1
  Transpose/1 -> Product1/1
  Direction Cosine Matrix to Rotation Angles/1 -> order-yaw_pitch_roll/1
  PS-Simulink Converter14/1 -> Quaternions to Direction Cosine Matrix/1
  PS-Simulink Converter17/1 -> Mux4/2
  PS-Simulink Converter19/1 -> Scope/1, Mux4/1
  PS-Simulink Converter18/1 -> Mux4/3
  Mux4/1 -> phi_sensing/1
  gimbal_command/1 -> MATLAB Function1/1(fd)
  MATLAB Function1/2(uav2) -> Demux/1
  MATLAB Function1/3(uav3) -> Demux2/1
  MATLAB Function1/4(uav4) -> Demux3/1
  MATLAB Function1/1(uav1) -> Demux1/1
  Demux1/1 -> Simulink-PS Converter/1
  Demux1/2 -> Simulink-PS Converter1/1
  Demux1/3 -> Simulink-PS Converter2/1
  Demux/3 -> Simulink-PS Converter5/1
  Demux/1 -> Simulink-PS Converter3/1
  Demux/2 -> Simulink-PS Converter4/1
  Demux2/3 -> Simulink-PS Converter8/1
  Demux2/1 -> Simulink-PS Converter7/1
  Demux2/2 -> Simulink-PS Converter9/1
  Demux3/3 -> Simulink-PS Converter11/1
  Demux3/1 -> Simulink-PS Converter6/1
  Demux3/2 -> Simulink-PS Converter12/1
  PS-Simulink Converter1/1 -> Quaternions to Direction Cosine Matrix1/1
  Quaternions to Direction Cosine Matrix1/1 -> fa2fb/1
  connections:
  Rigid Transform2/LConn1 -- Rigid Transform1/RConn1
  Mechanism Configuration/RConn1 -- Rigid Transform27/LConn1 -- 6-DOF Joint/LConn1 -- World Frame/RConn1 -- Solver Configuration/RConn1
  Rigid Transform18/LConn1 -- Rigid Transform9/RConn1
  Rigid Transform8/LConn1 -- Rigid Transform3/RConn1
  Rigid Transform24/LConn1 -- Rigid Transform19/RConn1
  PS-Simulink Converter8/LConn1 -- 6-DOF Joint/RConn2
  PS-Simulink Converter9/LConn1 -- 6-DOF Joint/RConn3
  PS-Simulink Converter10/LConn1 -- 6-DOF Joint/RConn4
  PS-Simulink Converter11/LConn1 -- 6-DOF Joint/RConn5
  PS-Simulink Converter12/LConn1 -- 6-DOF Joint/RConn6
  PS-Simulink Converter13/LConn1 -- 6-DOF Joint/RConn7
  PS-Simulink Converter14/LConn1 -- 6-DOF Joint/RConn8
  PS-Simulink Converter15/LConn1 -- 6-DOF Joint/RConn9
  Rigid Transform25/LConn1 -- 6-DOF Joint/RConn1
  Solid9/RConn1 -- Rigid Transform27/RConn1
  Rigid Transform25/RConn1 -- Cylindrical Solid/LConn1
  Rigid Transform9/LConn1 -- Rigid Transform1/LConn1 -- Rigid Transform26/LConn1 -- Cylindrical Solid1/RConn1
  Cylindrical Solid/RConn1 -- Rigid Transform/LConn1 -- Revolute Joint9/LConn1 -- Rigid Transform19/LConn1 -- Rigid Transform3/LConn1
  Cylindrical Solid1/LConn1 -- Revolute Joint9/RConn1
  Rigid Transform26/RConn1 -- Transform Sensor/LConn1
  Rigid Transform/RConn1 -- Transform Sensor/RConn1
  PS-Simulink Converter17/LConn1 -- Transform Sensor/RConn4
  Transform Sensor/RConn2 -- PS-Simulink Converter19/LConn1
  Transform Sensor/RConn5 -- PS-Simulink Converter18/LConn1
  External Force and Torque/RConn1 -- Rigid Transform24/RConn1
  External Force and Torque1/RConn1 -- Rigid Transform18/RConn1
  External Force and Torque2/RConn1 -- Rigid Transform8/RConn1
  External Force and Torque3/RConn1 -- Rigid Transform2/RConn1
  Simulink-PS Converter/RConn1 -- External Force and Torque/LConn1
  Simulink-PS Converter1/RConn1 -- External Force and Torque/LConn2
  Simulink-PS Converter2/RConn1 -- External Force and Torque/LConn3
  Simulink-PS Converter5/RConn1 -- External Force and Torque1/LConn3
  Simulink-PS Converter3/RConn1 -- External Force and Torque1/LConn1
  Simulink-PS Converter4/RConn1 -- External Force and Torque1/LConn2
  External Force and Torque2/LConn3 -- Simulink-PS Converter8/RConn1
  External Force and Torque2/LConn1 -- Simulink-PS Converter7/RConn1
  Simulink-PS Converter9/RConn1 -- External Force and Torque2/LConn2
  Simulink-PS Converter11/RConn1 -- External Force and Torque3/LConn3
  Simulink-PS Converter6/RConn1 -- External Force and Torque3/LConn1
  Simulink-PS Converter12/RConn1 -- External Force and Torque3/LConn2
  Transform Sensor/RConn3 -- PS-Simulink Converter1/LConn1

== matlab function simu_gimbal/girpper_controller ==
  data: phi input; M output; phi_desire input; K1 input; a input; Iz input; B input; K input
function M  =gripper_controller(phi,phi_desire,K1,a,Iz,B,K)

phi_error = (phi_desire(1)-phi(1));
phi_error_d = (phi_desire(2)-phi(2));
%phi_error_dd = (phi_desire(3)-phi(3));
r = phi_error_d + a*phi_error;
M = Iz*(B*phi(2)+K*phi(1))+Iz*phi_desire(3)+...
    Iz*K1*r-Iz*(a^2)*phi_error;
    
M = (M/2);

end

== matlab function simu_gimbal/MATLAB Function ==
  data: p input; u1 output; p_dot input; R input; pr input; pdr input; ep output; fr output; m parameter; epiout output; epiin input
function [u1, ep, fr, epiout] = position_controller(p, p_dot, R, pr, pdr, m, epiin)

% Kp = diag([8, 8, 5.35]);
% Kv = diag([6, 6, 3.54]);
% Ki = diag([0.2, 0.2, 0.05]);

% ucla provide gain
%Kp = diag([4.5, 4.5, 5]);
%Kv = diag([2,  2,  2.5]);
%Ki = diag([2.7, 2.5, 3]);

% my gain
 Kp = diag([10, 10, 25]);
 Kv = diag([2,  2,  2.5]);
 Ki = diag([0, 0, 0]);

ep = p - pr;
ev = p_dot - pdr;
epiout = epiin + ep*0.01;

% force in {I} frame
fr = m*(9.81*[0;0;1] - Kp*ep - Kv*ev - Ki*epiin);

% force in {B} frame
u1 = R.' * fr;

== matlab function simu_gimbal/Subsystem/MATLAB Function ==
  data: Rin input; Rout output
function Rout = y_coord_180(Rin)

% % y z reversed, x same
% Rout = diag([1,-1,-1])*Rin*diag([1,-1,-1]);

% all x y z reversed
Rout = Rin.';

== matlab function simu_gimbal/MATLAB Function1 ==
  data: R input; u2 output; O input; Rr input; agvr input; eR output; Lh parameter; m parameter; IB parameter; eRiin input; eRiout output; phi input; R_f2a input
function [u2, eR, eRiout] = attitude_controller(R, O, Rr, agvr, Lh, m, IB, eRiin,phi,R_f2a)

% KR = diag([17.07, 17.07, 17.07]);
% Kw = diag([6.65, 6.65, 6.65]);
% Ki = diag([6.41, 6.41, 6.41]);


% ucla provide gain
%KR = diag([5, 5, 8]);
%Kw = diag([6, 5.5, 3]);
%Ki = diag([5.5, 4.5 ,3]);



% my gain
 KR = diag([50, 25, 10]);
 Kw = diag([10, 5.5, 2.2]);
 Ki = diag([0, 0 ,0]);
J_A=[0,0,0;...
    0,3e-05,0;...
    0,0,3e-05];
J_F=[0,0,0;...
    0,3e-05,0;...
    0,0,3e-05];

S=[1,0,0;...
    0,1,0;...
    0,0,0];

R_F2A=R_f2a';
   
J_E = J_A+S*R_F2A'*J_F*R_F2A;

qc_mass_matrix=[0,0,0;...
               0,2*0.03,0;...
                0,0,2*0.03];

J_sys =J_E+(0.185^2)*qc_mass_matrix+S*R_F2A*(0.185^2)*qc_mass_matrix;

E = 1/2*(Rr.'*R - R.'*Rr);
eR = [E(3,2) E(1,3) E(2,1)]';
ew = O - R.'*(Rr*agvr);
eRiout = eRiin + eR*0.01;

% Physical dynamics to cancel
rho = Lh;
h = cross(O, J_E * O);
tau_g = - m * 9.81 * cross(rho, R.'*[0;0;1]);

u2 = h - tau_g - J_sys*(KR*eR + Kw*ew + Ki*eRiout);

== matlab function simu_gimbal/MATLAB Function2 ==
  data: u1 input; fd output; u2 input; Lw parameter; the input; M input; R_f2a input
function fd = wrench_mapper(u1, u2, Lw, the ,M,R_f2a)


%u2=[0;0;0];
%M = 5;




%Rotatiom matrix R_F2A

R_F2A=R_f2a';
   
%R_F2A=R_F2A';
%Rotation matrix F1 frame to F  frame
R_F12F = eye(3);

%Rotation matrix F2 frame to F  frame

R_F22F =[-1  0 0;  0 -1 0; 0 0 1];



BP1 = [ Lw   0  0]';%d_a1
BP2 = [ -Lw  0  0]';%d_a2
BP3 = [ Lw   0  0]'; %d_f1
BP4 = [ -Lw   0  0]';%d_f2


% bijection hat map
DA1x = [0,-BP1(3),BP1(2); BP1(3),0,-BP1(1); -BP1(2),BP1(1),0];  %DA1 
DA2x = [0,-BP2(3),BP2(2); BP2(3),0,-BP2(1); -BP2(2),BP2(1),0];  %DA2
DF1x = [0,-BP3(3),BP3(2); BP3(3),0,-BP3(1); -BP3(2),BP3(1),0];  %DF1
DF2x = [0,-BP4(3),BP4(2); BP4(3),0,-BP4(1); -BP4(2),BP4(1),0];  %DF2

% ===== skwe-symmetric can represent cross product ========
%tow vector cross product uxv = Su X v where Su is the skew-symmetric
%corresponding to the vector u
% =========================================================




% compile A matrix 
% Ar maps u to q expressed in {i}
%B1R = eye(3);
%B2R = [ 0 -1 0;  1  0 0; 0 0 1];

%B3R = [-1  0 0;  0 -1 0; 0 0 1];
%B4R = [ 0  1 0; -1  0 0; 0 0 1];

% The first line for W matrix

R_A12A=eye(3);
R_A22A=[-1  0 0;  0 -1 0; 0 0 1];
R_F12A=R_F2A*R_F12F;
R_F22A=R_F2A*R_F22F;


%Ar = A * [B1R,zeros(3,9); zeros(3,3),B2R,zeros(3,6); zeros(3,6),B3R,zeros(3,3); zeros(3,9),B4R];
%Ar =[Ar;BP1x*B1R,zeros(3,3),BP3x*B3R,zeros(3,3);zeros(3,3),BP2x*B2R,zeros(3,3),BP4x*B4R];
% on the paper Ar is W,Art is pseude inverse of A

%======== additional control input constraints========%
W1 =[0 0 1]*DA1x*R_A12A;
W2 =[0 0 -1]*DF1x*R_F12F;
W3 =[0 0 1]*DA2x*R_A22A;
W4 =[0 0 -1]*DF2x*R_F22F;
%Ar = [Ar;W1,W2,W3,W4];


Ar=[R_A12A,R_F12A,R_A22A,R_F22A;...
    DA1x*R_A12A,R_F2A*DF1x*R_F12F,DA2x*R_A22A,R_F2A*R_F2A*DF2x*R_F22F;...
    W1,W2,W3,W4];


% =========================================%
ArT = Ar.'*((Ar*Ar.')^(-1));
%fd = ArT * [u1;u2;M1-M2];
fd = ArT * [u1;u2;M];

end

== matlab function simu_gimbal/Subsystem/MATLAB Function1 ==
  data: fd input; uav1 output; uav2 output; uav3 output; uav4 output
function [uav1,uav2,uav3,uav4] = platform_force(fd)




uav1 =[fd(1),fd(2),fd(3)];
uav2 =[fd(4),fd(5),fd(6)];
uav3 =[fd(7),fd(8),fd(9)];
uav4 =[fd(10),fd(11),fd(12)];

== matlab function simu_gimbal/MATLAB Function4 ==
  data: pr output; t input; Rr output; StepSize parameter; pdr output; agvr output; rpyr output; rpyr_prev input; phi_desire output
function [pr, Rr, pdr, agvr, rpyr,phi_desire] = program_trajectory(t,StepSize, rpyr_prev)

MODE_SELECT = 6;  %use the to choice trojectory
dt = StepSize;

pr = [0;0;0];
rpyr = [0;0;0];
pdr = [0;0;0];
agvr = [0;0;0];

phid = deg2rad(120);
phid_d = 0;
phid_dd = 0;

% % %%%%%%%%% CHOOSE ONE CONFIG BELOW %%%%%%%%%%%%%

switch MODE_SELECT

    case 1
%% ===== 360 deg rotation configuration ===== %%
    A = [0, 0, -pi/2, -pi/2, -pi, -pi, -pi*2, -pi*2];
    t1 = [0,0.01,    8,     3,   8,   3,    12,   100];
    frag = 1;
    for i=1:length(t1)
        if t >= sum(t1(1:i))
            frag = frag+1;
        else
            break;
        end
    w = 2*pi/t1(frag)*1/2;
    tnow = t - sum(t1(1:(frag-1)));

    As = A(frag-1); Ag = A(frag);

    rpyr(2) = (Ag-As)/2 - (Ag-As)/2*cos(w*tnow) + As;
    agvr(2) = (Ag-As)/2*w*sin(w*tnow);
    end

    case 2
%% ===== normal 6DOF configuration ===== %%
tinit = 0.5;
%trajectory for paper
Apos = [0.3, -0.4, 0.3];
Arpy = [-0.4, 0.4, 1];
tpos1 = [20, 16, 30];
tpos2 = [100, 100, 100];
trpy1 = [7, 7, 14];
trpy2 = [4, 4, 9];
wpos = 2*pi./tpos1*1/2;
wrpy = 2*pi./trpy1*1/2;


  if t >= tinit
    t = t-tinit;
   % ======= design desire q1 and q2 ======== %
    phid = 0.4*sin(t)+deg2rad(90);
    phid_d = 0.4*cos(t);
    phid_dd = -0.4*sin(t);
        
    
    
    for i=1:3
        pr(i) = current_pos(Apos(i), wpos(i), t, tpos1(i), tpos2(i));
        pdr(i) = current_vel(Apos(i), wpos(i), t, tpos1(i), tpos2(i));
        rpyr(i) = current_pos(Arpy(i), wrpy(i), t, trpy1(i), trpy2(i));
        agvr(i) = current_vel(Apos(i), wpos(i), t, tpos1(i), tpos2(i));
    end
end
    case 3
 %% ===== cross configuration ===== %%
% parameters of cross
    tc = 15;
    Ac = pi/2;
    wc = 2*pi/tc*1/2;
    if t <= tc
        thetac = Ac/2-Ac/2*cos(wc*t);
    else
        thetac = Ac/2-Ac/2*cos(wc*tc);
    end
    q0=cos(thetac/2);q1=sin(thetac/2)/sqrt(2);q2=sin(thetac/2)/sqrt(2);q3=0;
    rpyr(1) = atan2(2*(q0*q1+q2*q3),1-2*(q1^2+q2^2));
    rpyr(2) = asin(2*(q0*q2-q3*q1));
    rpyr(3) = atan2(2*(q0*q3+q1*q2),1-2*(q2^2+q3^2));
    agvr = (rpyr - rpyr_prev) / 0.002;

    

   



    case 4
%% ===== radious motion heading not change ====%%
    % ===== platform trajectory ==== %
    r = 1 ; %radius
    p = 10 ;  %period
    theta = (2*pi)/p;
    
    pr = [r*cos(t*theta) ; r*sin(t*theta) ; 0];
    pdr = [-r*theta*sin(t*theta) ; r*theta*cos(t*theta) ;0];
    
    rpyr = [0;0;0];  %attitude not change
    agvr = [0;0;0];  % omega is 0
    
    % ===== gripper motion ===== %
   % phid = 0.4*sin(t)+deg2rad(90);
    %phid_d = 0.4*cos(t);
   % phid_dd = -0.4*sin(t);
   phid = deg2rad(120);
phid_d = 0;
phid_dd = 0;
    
    case 5
%% ====== radious motion heading change ====%%
    r = 1;%radius
    p = 10; %period
    theta = (2*pi)/p;
    % translation
    pr = [r*cos(t*theta) ; r*sin(t*theta) ; 0];
    pdr = [-r*theta*sin(t*theta) ; r*theta*cos(t*theta) ;0];
    %rotation
    rpyr = [0;0;t*theta];
    agvr = [0;0;theta];
        % ===== gripper motion ===== %
    phid = 0.4*sin(t)+deg2rad(90);
    phid_d = 0.4*cos(t);
    phid_dd = -0.4*sin(t);

    
    
end
    
phi_desire = [phid,phid_d,phid_dd];

Rx = [1 0 0; 0 cos(rpyr(1)) -sin(rpyr(1)); 0 sin(rpyr(1)) cos(rpyr(1))];
Ry = [cos(rpyr(2)) 0 sin(rpyr(2)); 0 1 0; -sin(rpyr(2)) 0 cos(rpyr(2))];
Rz = [cos(rpyr(3)) -sin(rpyr(3)) 0; sin(rpyr(3)) cos(rpyr(3)) 0; 0 0 1];
Rr = Rz * Ry * Rx;
